simulink model "Attitude_Tracking_Test"  (R2017b)
settings: Solver=VariableStepAuto  StartTime=0.0  StopTime=10.0  RelTol=1e-3
undefined symbols (not defined in the file): IC, quadModel
libraries: NLGCToolbox x5, simulink x5
settings Model: Creator=hoang  LastModifiedBy=hoang

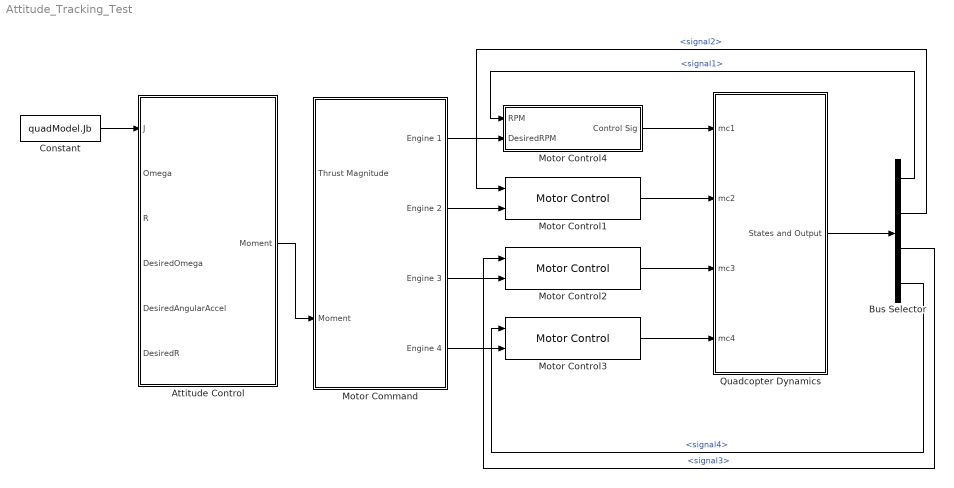
== system Attitude_Tracking_Test ==
  Attitude Control : Subsystem  mask{kr=96, ko=1.25}
      mask prompts: kr "Attitude error gain (Kr)"; ko "Angular velocity error gain (Ko)"
      mask init:
      | set_param(gcb, 'MaskSelfModifiable', 'on');
      settings: OpenFcn=set_param(gcbh,'LinkStatus','none');
  Bus Selector : BusSelector  OutputSignals=mc and RPM.signal1,mc and RPM.signal2,mc and RPM.signal3,mc and RPM.signal4
  Constant : Constant  Value=quadModel.Jb
  Motor Command : Subsystem  mask{Ct=quadModel.ct, dctcq=quadModel.dctcq}
      mask prompts: Ct "Force coefficient (Ct)"; dctcq "Moment coefficients (dctcq)"
      settings: OpenFcn=set_param(gcbh,'LinkStatus','none');
  Motor Control1 : NLGCToolbox/Motor Control  k=2.26  Km=quadModel.cr  Ts=1/60  T=quadModel.T  Rdt=100  Rdx=2  b=quadModel.b
      settings: SourceProductName=Thinh - NLGC for Quadrotor
  Motor Control2 : NLGCToolbox/Motor Control  k=2.26  Km=quadModel.cr  Ts=1/60  T=quadModel.T  Rdt=100  Rdx=2  b=quadModel.b
      settings: SourceProductName=Thinh - NLGC for Quadrotor
  Motor Control3 : NLGCToolbox/Motor Control  k=2.26  Km=quadModel.cr  Ts=1/60  T=quadModel.T  Rdt=100  Rdx=2  b=quadModel.b
      settings: SourceProductName=Thinh - NLGC for Quadrotor
  Motor Control4 : Subsystem  mask{k=2.26, Km=quadModel.cr, Ts=1/60, T=quadModel.T, Rdt=100, Rdx=2, b=quadModel.b}
      mask prompts: k "Velocity Gain (k)"; Km "Motor Amplification (Km)"; Ts "Sampling Time (Ts)"; T "Motor Time Constant (T)"; Rdt "Maximum Output Threshold (Rdt)"; Rdx "Maximum Derivative Threshold (Rdx)"; b "Throttle Bias"
      settings: OpenFcn=set_param(gcbh,'LinkStatus','none');
  Quadcopter Dynamics : Subsystem
  wires:
  Constant/1 -> Attitude Control/1(J)
  Attitude Control/1(Moment) -> Motor Command/2(Moment)
  Motor Command/1(Engine 1) -> Motor Control4/2(DesiredRPM)
  Motor Command/2(Engine 2) -> Motor Control1/2
  Motor Command/3(Engine 3) -> Motor Control2/2
  Motor Command/4(Engine 4) -> Motor Control3/2
  Motor Control3/1 -> Quadcopter Dynamics/4(mc4)
  Motor Control2/1 -> Quadcopter Dynamics/3(mc3)
  Motor Control1/1 -> Quadcopter Dynamics/2(mc2)
  Motor Control4/1(Control Sig) -> Quadcopter Dynamics/1(mc1)
  Quadcopter Dynamics/1(States and Output) -> Bus Selector/1
  Bus Selector/1 -> Motor Control4/1(RPM)  "<signal1>"
  Bus Selector/2 -> Motor Control1/1  "<signal2>"
  Bus Selector/3 -> Motor Control2/1  "<signal3>"
  Bus Selector/4 -> Motor Control3/1  "<signal4>"

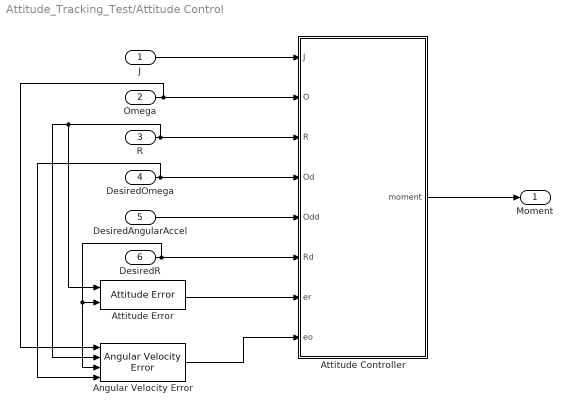
== system Attitude_Tracking_Test/Attitude Control ==
  J : Inport
  Omega : Inport  Port=2
  R : Inport  Port=3
  DesiredOmega : Inport  Port=4
  DesiredAngularAccel : Inport  Port=5
  DesiredR : Inport  Port=6
  Angular Velocity Error : NLGCToolbox/Angular Velocity Error
      settings: SourceProductName=Thinh - NLGC for Quadrotor
  Attitude Controller : MATLAB Function  TreatAsAtomicUnit=on
  Attitude Error : NLGCToolbox/Attitude Error
      settings: SourceProductName=Thinh - NLGC for Quadrotor
  Moment : Outport
  wires:
  Angular Velocity Error/1 -> Attitude Controller/8(eo)
  Attitude Error/1 -> Attitude Controller/7(er)
  J/1 -> Attitude Controller/1(J)
  Omega/1 -> Attitude Controller/2(O), Angular Velocity Error/1
  R/1 -> Attitude Controller/3(R), Angular Velocity Error/2, Attitude Error/1
  DesiredOmega/1 -> Attitude Controller/4(Od), Angular Velocity Error/4
  DesiredAngularAccel/1 -> Attitude Controller/5(Odd)
  DesiredR/1 -> Attitude Controller/6(Rd), Attitude Error/2, Angular Velocity Error/3
  Attitude Controller/1(moment) -> Moment/1

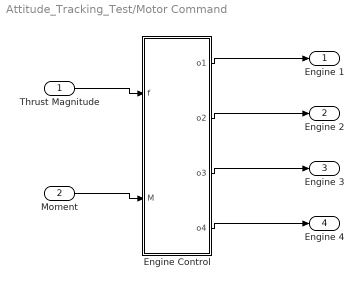
== system Attitude_Tracking_Test/Motor Command ==
  " Thrust Magnitude" : Inport
  Moment : Inport  Port=2
  Engine Control : MATLAB Function  TreatAsAtomicUnit=on
  Engine 1 : Outport
  Engine 2 : Outport  Port=2
  Engine 3 : Outport  Port=3
  Engine 4 : Outport  Port=4
  wires:
  Engine Control/4(o4) -> Engine 4/1
  Engine Control/3(o3) -> Engine 3/1
  Engine Control/2(o2) -> Engine 2/1
  Engine Control/1(o1) -> Engine 1/1
  Moment/1 -> Engine Control/2(M)
  " Thrust Magnitude"/1 -> Engine Control/1(f)

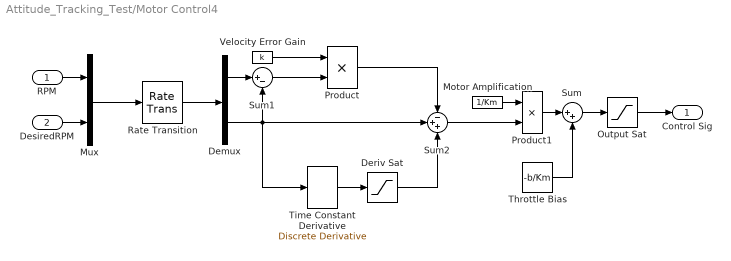
== system Attitude_Tracking_Test/Motor Control4 ==
  RPM : Inport
  DesiredRPM : Inport  Port=2
  Demux : Demux  Outputs=2
  Deriv Sat : Saturate  UpperLimit=Rdx  LowerLimit=-Rdx
  Motor Amplification : Constant  Value=1/Km
  Mux : Mux  Inputs=2
  Output Sat : Saturate  UpperLimit=Rdt  LowerLimit=0
  Product : Product
  Product1 : Product
  Rate Transition : RateTransition  OutPortSampleTime=Ts
  Sum : Sum  Inputs=|++
  Sum1 : Sum  Inputs=|+-
  Sum2 : Sum  Inputs=-++
  Throttle Bias : Constant  Value=-b/Km
  Time Constant Derivative : simulink/Discrete/Discrete Derivative  gainval=T  ICPrevScaledInput=0.0  OutMin=[]  OutMax=[]  OutDataType=fixdt(1, 16)  OutScaling=2^-10  DoSatur=off
  Velocity Error Gain : Constant  Value=k
  Control Sig : Outport
  wires:
  Throttle Bias/1 -> Sum/2
  Sum/1 -> Output Sat/1
  Product1/1 -> Sum/1
  Deriv Sat/1 -> Sum2/3
  Time Constant Derivative/1 -> Deriv Sat/1
  Output Sat/1 -> Control Sig/1
  Motor Amplification/1 -> Product1/1
  Sum2/1 -> Product1/2
  Product/1 -> Sum2/1
  Velocity Error Gain/1 -> Product/1
  Sum1/1 -> Product/2
  Demux/1 -> Sum1/1
  Demux/2 -> Sum1/2, Sum2/2, Time Constant Derivative/1
  Rate Transition/1 -> Demux/1
  Mux/1 -> Rate Transition/1
  DesiredRPM/1 -> Mux/2
  RPM/1 -> Mux/1

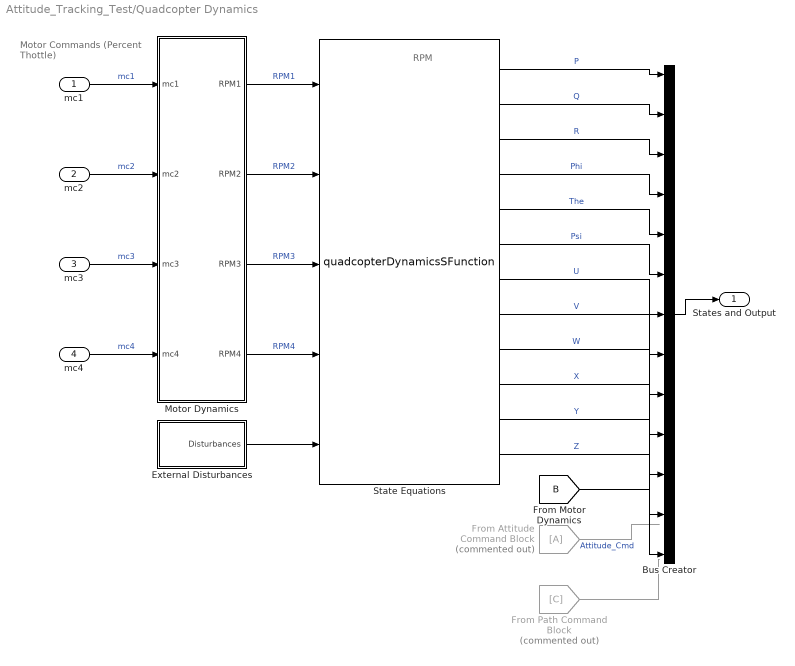
== system Attitude_Tracking_Test/Quadcopter Dynamics ==
  note: RPM
  note: Motor Commands
      | (Percent Thottle)
  mc1 : Inport
  mc2 : Inport  Port=2
  mc3 : Inport  Port=3
  mc4 : Inport  Port=4
  Bus Creator : BusCreator  Inputs=P,Q,R,Phi,The,Psi,U,V,W,X,Y,Z,mc and RPM
  External Disturbances : Subsystem
  From Attitude Command Block : From  Commented=on  TagVisibility=global
  From Path Command Block : From  Commented=on  GotoTag=C  TagVisibility=global
  Motor Dynamics : Subsystem
  State Equations : M-S-Function  FunctionName=quadcopterDynamicsSFunction  Parameters=quadModel, IC
      mask Display:
      | port_label('input', 1, 'RPM1')
      | port_label('input', 2, 'RPM2')
      | port_label('input', 3, 'RPM3')
      | port_label('input', 4, 'RPM4')
      | port_label('input', 5, 'Disturbances')
      | port_label('output', 1, 'P')
      | port_label('output', 2, 'Q')
      | port_label('output', 3, 'R')
      | port_label('output', 4, 'Phi')
      | port_label('output', 5, 'The')
      | port_label('output', 6, 'Psi')
      | port_label('output', 7, 'U')
      | port_label('output', 8, 'V')
      | port_label('output', 9, 'W')
      | port_label('output', 10, 'X')
      | port_label('output', 11, 'Y')
      | port_label('output', 12, 'Z')
  States and Output : Outport
  wires:
  State Equations/1 -> Bus Creator/1  "P"
  State Equations/2 -> Bus Creator/2  "Q"
  State Equations/3 -> Bus Creator/3  "R"
  State Equations/4 -> Bus Creator/4  "Phi"
  State Equations/5 -> Bus Creator/5  "The"
  State Equations/6 -> Bus Creator/6  "Psi"
  State Equations/7 -> Bus Creator/7  "U"
  State Equations/8 -> Bus Creator/8  "V"
  State Equations/9 -> Bus Creator/9  "W"
  State Equations/10 -> Bus Creator/10  "X"
  State Equations/11 -> Bus Creator/11  "Y"
  State Equations/12 -> Bus Creator/12  "Z"
  Bus Creator/1 -> States and Output/1
  Motor Dynamics/1(RPM1) -> State Equations/1  "RPM1"
  Motor Dynamics/2(RPM2) -> State Equations/2  "RPM2"
  Motor Dynamics/3(RPM3) -> State Equations/3  "RPM3"
  Motor Dynamics/4(RPM4) -> State Equations/4  "RPM4"
  mc1/1 -> Motor Dynamics/1(mc1)  "mc1"
  mc4/1 -> Motor Dynamics/4(mc4)  "mc4"
  mc3/1 -> Motor Dynamics/3(mc3)  "mc3"
  mc2/1 -> Motor Dynamics/2(mc2)  "mc2"
  External Disturbances/1("Disturbances ") -> State Equations/5
  From Attitude Command Block/1 -> ?  "Attitude_Cmd"
  [B] -> Bus Creator/13
  From Path Command Block/1 -> ?

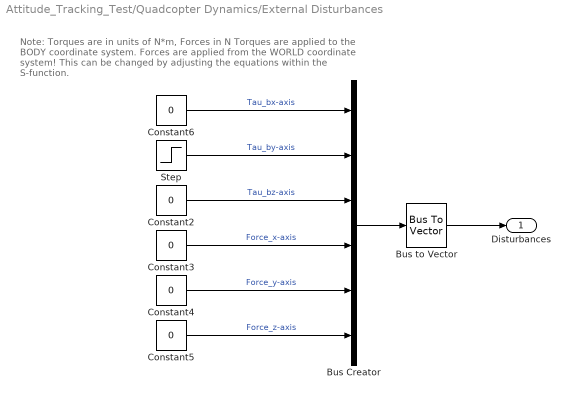
== system Attitude_Tracking_Test/Quadcopter Dynamics/External Disturbances ==
  note: Note: Torques are in units of N*m, Forces in N
      | Torques are applied to the BODY coordinate system.
      | Forces are applied from the WORLD coordinate system!
      | This can be changed by adjusting the equations within the S-function.
  Bus Creator : BusCreator  Inputs=6
  Bus to Vector : BusToVector
  Constant{2..6} (5 alike) : Constant  Value=0
  Step : Step  After=0  SampleTime=0
  "Disturbances " : Outport
  wires:
  Bus to Vector/1 -> "Disturbances "/1
  Bus Creator/1 -> Bus to Vector/1
  Constant6/1 -> Bus Creator/1  "Tau_bx-axis"
  Step/1 -> Bus Creator/2  "Tau_by-axis"
  Constant2/1 -> Bus Creator/3  "Tau_bz-axis"
  Constant3/1 -> Bus Creator/4  "Force_x-axis"
  Constant4/1 -> Bus Creator/5  "Force_y-axis"
  Constant5/1 -> Bus Creator/6  "Force_z-axis"

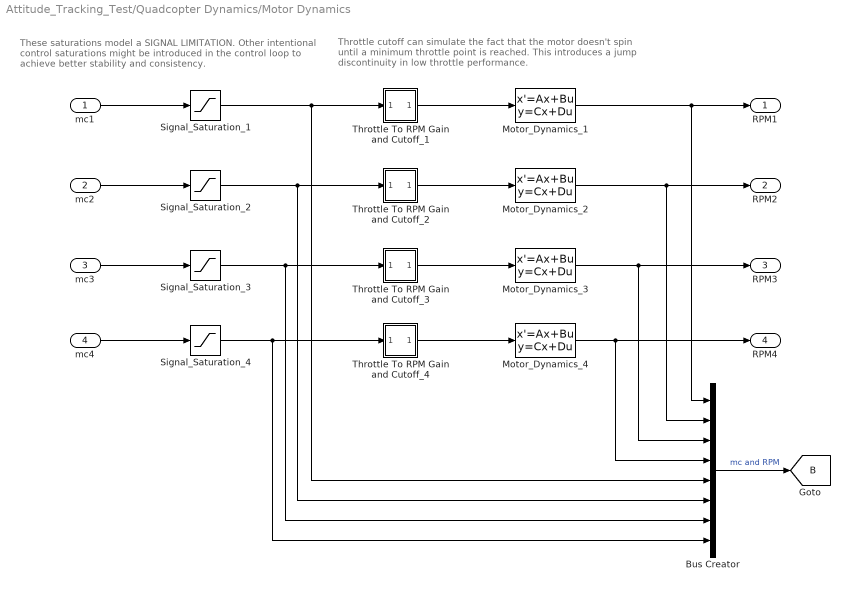
== system Attitude_Tracking_Test/Quadcopter Dynamics/Motor Dynamics ==
  note: Throttle cutoff can simulate the fact that the motor doesn't
      | spin until a minimum throttle point is reached. This introduces
      | a jump discontinuity in low throttle performance.
  note: These saturations model a SIGNAL LIMITATION.
      | Other intentional control saturations might be introduced in the
      | control loop to achieve better stability and consistency.
  mc1 : Inport
  mc2 : Inport  Port=2
  mc3 : Inport  Port=3
  mc4 : Inport  Port=4
  Bus Creator : BusCreator  Inputs=8
  Motor_Dynamics_1 : StateSpace  A=-1/quadModel.T  C=1/quadModel.T  D=0  InitialCondition=IC.w1*quadModel.T
  Motor_Dynamics_2 : StateSpace  A=-1/quadModel.T  C=1/quadModel.T  D=0  InitialCondition=IC.w2*quadModel.T
  Motor_Dynamics_3 : StateSpace  A=-1/quadModel.T  C=1/quadModel.T  D=0  InitialCondition=IC.w3*quadModel.T
  Motor_Dynamics_4 : StateSpace  A=-1/quadModel.T  C=1/quadModel.T  D=0  InitialCondition=IC.w4*quadModel.T
  Signal_Saturation_{1..4} (4 alike) : Saturate  UpperLimit=100  LowerLimit=0
  Throttle To RPM Gain and Cutoff_1 : Subsystem
  Throttle To RPM Gain and Cutoff_2 : Subsystem
  Throttle To RPM Gain and Cutoff_3 : Subsystem
  Throttle To RPM Gain and Cutoff_4 : Subsystem
  RPM1 : Outport
  RPM2 : Outport  Port=2
  RPM3 : Outport  Port=3
  RPM4 : Outport  Port=4
  tag scope: B=global
  wires:
  mc1/1 -> Signal_Saturation_1/1
  mc4/1 -> Signal_Saturation_4/1
  mc2/1 -> Signal_Saturation_2/1
  mc3/1 -> Signal_Saturation_3/1
  Signal_Saturation_1/1 -> Bus Creator/5, Throttle To RPM Gain and Cutoff_1/1(In5)
  Signal_Saturation_2/1 -> Bus Creator/6, Throttle To RPM Gain and Cutoff_2/1(In5)
  Signal_Saturation_3/1 -> Bus Creator/7, Throttle To RPM Gain and Cutoff_3/1(In5)
  Signal_Saturation_4/1 -> Bus Creator/8, Throttle To RPM Gain and Cutoff_4/1(In5)
  Throttle To RPM Gain and Cutoff_1/1(Out5) -> Motor_Dynamics_1/1
  Throttle To RPM Gain and Cutoff_2/1(Out5) -> Motor_Dynamics_2/1
  Throttle To RPM Gain and Cutoff_3/1(Out5) -> Motor_Dynamics_3/1
  Throttle To RPM Gain and Cutoff_4/1(Out5) -> Motor_Dynamics_4/1
  Motor_Dynamics_1/1 -> Bus Creator/1, RPM1/1
  Motor_Dynamics_2/1 -> Bus Creator/2, RPM2/1
  Motor_Dynamics_3/1 -> Bus Creator/3, RPM3/1
  Motor_Dynamics_4/1 -> Bus Creator/4, RPM4/1
  Bus Creator/1 -> [B]  "mc and RPM"

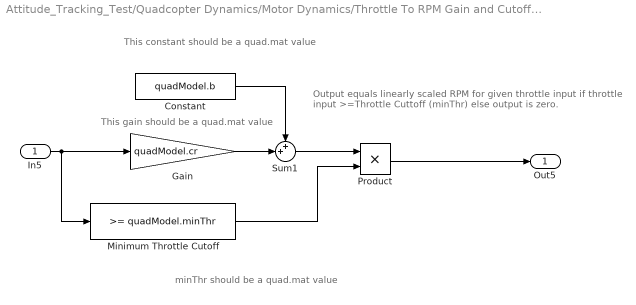
== system Attitude_Tracking_Test/Quadcopter Dynamics/Motor Dynamics/Throttle To RPM Gain and Cutoff_1 ==
  note: minThr should be a quad.mat value
  note: This gain should be a quad.mat value
  note: This constant should be a quad.mat value
  note: Output equals linearly scaled RPM
      | for given throttle input if throttle input >=Throttle Cuttoff (minThr)
      | else output is zero.
  In5 : Inport
  Constant : Constant  Value=quadModel.b
  Gain : Gain  Gain=quadModel.cr
  Minimum Throttle Cutoff : simulink/Logic and Bit Operations/Compare To Constant  relop=>=  const=quadModel.minThr  OutDataTypeStr=uint8
  Product : Product
  Sum1 : Sum  Inputs=++|
  Out5 : Outport
  wires:
  Minimum Throttle Cutoff/1 -> Product/2
  Product/1 -> Out5/1
  In5/1 -> Gain/1, Minimum Throttle Cutoff/1
  Gain/1 -> Sum1/2
  Sum1/1 -> Product/1
  Constant/1 -> Sum1/1

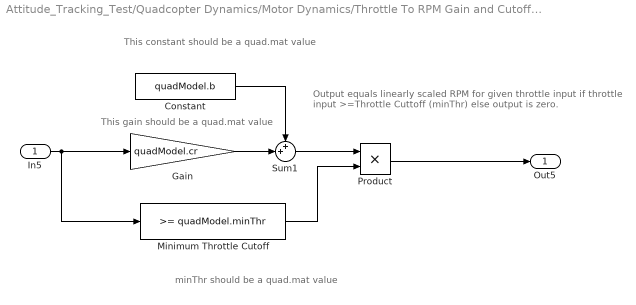
== system Attitude_Tracking_Test/Quadcopter Dynamics/Motor Dynamics/Throttle To RPM Gain and Cutoff_2 ==
  note: minThr should be a quad.mat value
  note: This gain should be a quad.mat value
  note: This constant should be a quad.mat value
  note: Output equals linearly scaled RPM
      | for given throttle input if throttle input >=Throttle Cuttoff (minThr)
      | else output is zero.
  In5 : Inport
  Constant : Constant  Value=quadModel.b
  Gain : Gain  Gain=quadModel.cr
  Minimum Throttle Cutoff : simulink/Logic and Bit Operations/Compare To Constant  relop=>=  const=quadModel.minThr  OutDataTypeStr=uint8
  Product : Product
  Sum1 : Sum  Inputs=++|
  Out5 : Outport
  wires:
  Minimum Throttle Cutoff/1 -> Product/2
  Product/1 -> Out5/1
  In5/1 -> Gain/1, Minimum Throttle Cutoff/1
  Gain/1 -> Sum1/2
  Sum1/1 -> Product/1
  Constant/1 -> Sum1/1

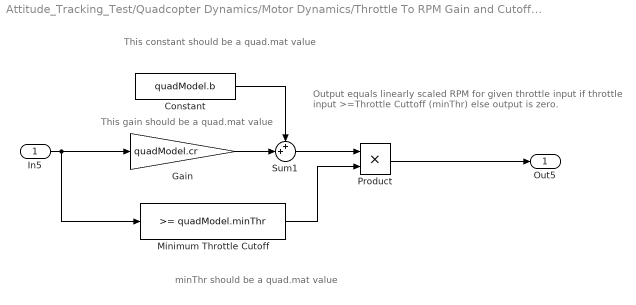
== system Attitude_Tracking_Test/Quadcopter Dynamics/Motor Dynamics/Throttle To RPM Gain and Cutoff_3 ==
  note: minThr should be a quad.mat value
  note: This gain should be a quad.mat value
  note: This constant should be a quad.mat value
  note: Output equals linearly scaled RPM
      | for given throttle input if throttle input >=Throttle Cuttoff (minThr)
      | else output is zero.
  In5 : Inport
  Constant : Constant  Value=quadModel.b
  Gain : Gain  Gain=quadModel.cr
  Minimum Throttle Cutoff : simulink/Logic and Bit Operations/Compare To Constant  relop=>=  const=quadModel.minThr  OutDataTypeStr=uint8
  Product : Product
  Sum1 : Sum  Inputs=++|
  Out5 : Outport
  wires:
  Minimum Throttle Cutoff/1 -> Product/2
  Product/1 -> Out5/1
  In5/1 -> Gain/1, Minimum Throttle Cutoff/1
  Gain/1 -> Sum1/2
  Sum1/1 -> Product/1
  Constant/1 -> Sum1/1

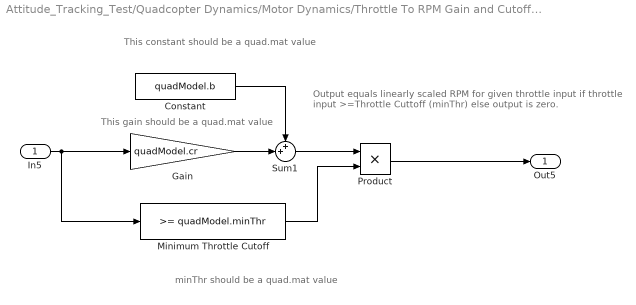
== system Attitude_Tracking_Test/Quadcopter Dynamics/Motor Dynamics/Throttle To RPM Gain and Cutoff_4 ==
  note: minThr should be a quad.mat value
  note: This gain should be a quad.mat value
  note: This constant should be a quad.mat value
  note: Output equals linearly scaled RPM
      | for given throttle input if throttle input >=Throttle Cuttoff (minThr)
      | else output is zero.
  In5 : Inport
  Constant : Constant  Value=quadModel.b
  Gain : Gain  Gain=quadModel.cr
  Minimum Throttle Cutoff : simulink/Logic and Bit Operations/Compare To Constant  relop=>=  const=quadModel.minThr  OutDataTypeStr=uint8
  Product : Product
  Sum1 : Sum  Inputs=++|
  Out5 : Outport
  wires:
  Minimum Throttle Cutoff/1 -> Product/2
  Product/1 -> Out5/1
  In5/1 -> Gain/1, Minimum Throttle Cutoff/1
  Gain/1 -> Sum1/2
  Sum1/1 -> Product/1
  Constant/1 -> Sum1/1

== matlab function Attitude_Tracking_Test/Attitude Control/Attitude Controller ==
  data: J input size=[3 3]; moment output size=[3 1]; O input size=[3 1]; R input size=[3 3]; Od input size=[3 1]; Odd input size=[3 1]; Rd input size=[3 3]; er input size=[3 1]; eo input size=[3 1]; kr parameter; ko parameter
function moment = fcn(J,O,R,Od,Odd,Rd,er,eo,kr, ko)
moment = hat(O)*(J*O) - J*(hat(O)*R'*Rd*Od - R'*Rd*Odd + kr * er + ko * eo);

== matlab function Attitude_Tracking_Test/Motor Command/Engine Control ==
  data: f input size=1; o1 output size=1; M input size=[3 1]; o2 output size=1; o3 output size=1; o4 output size=1; Ct parameter; dctcq parameter size=[3 4]
function [o1,o2,o3,o4] = fcn(f,M,Ct,dctcq)
force = [f; M];
gamma = [Ct Ct Ct Ct; dctcq];
omega_sq = gamma\force;
if(omega_sq>0)
    omega = sqrt(gamma\force);
else
    omega = [0 0 0 0]';
end
o1=omega(1);
o2=omega(2);
o3=omega(3);
o4=omega(4);
1+1;
